simulink model "EKF_SPM_Slx2019"  (R2019a)
settings: Solver=ode45  StartTime=0.0  StopTime=0.7  MaxStep=5e-6  RelTol=1e-3
values from neighbouring files (symbols this model uses):
  alpha = 2*pi*200    (= 1256.63706144)    [EKF_SPM_settings.m]
  alphas = log(9)/t_rc    [EKF_SPM_settings.m]
  d = [-1/Ld; 0]    [EKF_SPM_settings.m]
  fpwm = 20e3    (= 20000)    [EKF_SPM_settings.m]
  gainAngle_noise = 0    [EKF_SPM_settings.m]
  gainSpeed_noise = 3.6 /60*2*pi    (= 0.376991118431)    [EKF_SPM_settings.m]
  inertia = 1.8e-4    (= 0.00018)    [EKF_SPM_settings.m]
  ivar = istdDev^2    (= 11.6508444444)    [EKF_SPM_settings.m]
  J = skewdec(2,0)    [EKF_SPM_settings.m]
  Kbs = 2/Kp_speed    [EKF_SPM_settings.m]
  ki = (-5.135 + 5.347)/Ts    (= 4240)    [EKF_SPM_settings.m]
  Ki_speed = (alphas/2/zeta)^2*inertia    [EKF_SPM_settings.m]
  kp = 5.347    [EKF_SPM_settings.m]
  Kp_speed = alphas*inertia    [EKF_SPM_settings.m]
  Ld = 3e-3    (= 0.003)    [EKF_SPM_settings.m]
  Linv = inv(L)    [EKF_SPM_settings.m]
  Lq = 3e-3    (= 0.003)    [EKF_SPM_settings.m]
  LT = 2.8    [EKF_SPM_settings.m]
  m = 3    [EKF_SPM_settings.m]
  p = 4    [EKF_SPM_settings.m]
  P0 = diag([0.1 0.1 200 10])    [EKF_SPM_settings.m]
  phi_PM = 0.1    [EKF_SPM_settings.m]
  Q = eye(4)    [EKF_SPM_settings.m]
  Qd = eye(4)    [EKF_SPM_settings.m]
  R = 1.9    [EKF_SPM_settings.m]
  R_cov = meas_sd^2*eye(2)    [EKF_SPM_settings.m]
  ramp_rate = 5    [EKF_SPM_settings.m]
  Rs = R    (= 1.9)    [EKF_SPM_settings.m]
  seed_1 = round(rand*(2^32-1))    [EKF_SPM_settings.m]
  seed_2 = round(rand*(2^32-1))    [EKF_SPM_settings.m]
  seed_4 = round(rand*(2^32-1))    [EKF_SPM_settings.m]
  seed_5 = round(rand*(2^32-1))    [EKF_SPM_settings.m]
  seed_6 = round(rand*(2^32-1))    [EKF_SPM_settings.m]
  snoise_mean = 0    [EKF_SPM_settings.m]
  snoise_std = 0.5    [EKF_SPM_settings.m]
  Ts = 1/fpwm    (= 5e-05)    [EKF_SPM_settings.m]
  Tspeed = Ts*10/10    (= 5e-05)    [EKF_SPM_settings.m]
  Vdc = 450    [EKF_SPM_settings.m]
  wm = 2*pi*ff    (= 1675.51608191)    [EKF_SPM_settings.m]
  zeta = 0.9    [EKF_SPM_settings.m]
undefined symbols (not defined in the file or in its folder): ssensor
libraries: simulink x11
(part 1 of 2)
settings Model: Creator=Nicky  LastModifiedBy=b6055800
settings DebuggingCC: ArithmeticOperatorsInVariantConditions=warning
settings CodeAppCC: StateflowObjectComments=on

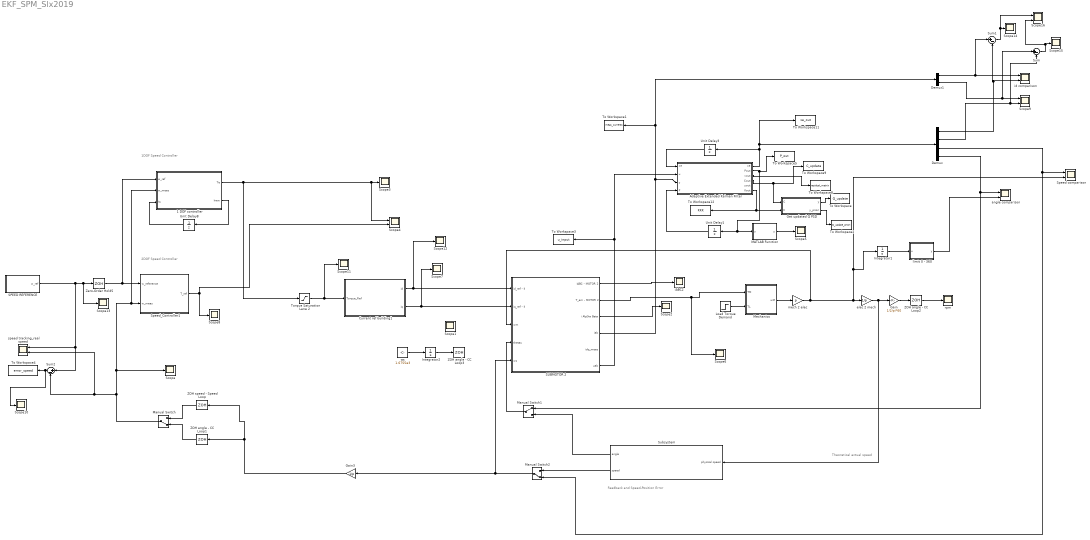
== system EKF_SPM_Slx2019 ==
  note: Theoretical actual speed
  note: Feedback and Speed-Position Error
  note: 2DOF Speed Controller
  note: 1DOF Speed Controller
  1 DOF controller : MATLAB Function  TreatAsAtomicUnit=on
  Adaptive Extended Kalman Filter : MATLAB Function  TreatAsAtomicUnit=on
  Current ref building1 : Subsystem
  Demux : Demux
  Demux1 : Demux  Outputs=2
  Gain : Gain  Gain=1/2/pi*60
  Gain3 : Gain  Gain=1/p
  Get updated Q PSD : MATLAB Function  TreatAsAtomicUnit=on
  Integrator1 : Integrator
  Integrator2 : Integrator
  Load Torque Demand : Step  Time=0.4  After=LT  SampleTime=0
  MATLAB Function : MATLAB Function  TreatAsAtomicUnit=on
  Manual Switch : ManualSwitch  CurrentSetting=0
  Manual Switch1 : ManualSwitch
  Manual Switch2 : ManualSwitch  CurrentSetting=0
  Mechanics : Subsystem
  "SPEED REFERENCE " : Subsystem
  SUBMOTOR 2 : Subsystem
  Scope{,1..3,5..8,10..15} (14 alike) : Scope
  Scope16 : Scope  NumInputPorts=2
  Scope4 : Scope  NumInputPorts=2
  Scope9 : Scope  NumInputPorts=2
  Speed comparison : Scope  NumInputPorts=2
  Speed_Controller1 : Subsystem
  Subsystem : Subsystem
  Sum : Sum  Inputs=|+-
  Sum1 : Sum  Inputs=|+-
  Sum2 : Sum  Inputs=|+-
  To Workspace : ToWorkspace  VariableName=Q_update  SaveFormat=Timeseries  SampleTime=-1
  To Workspace1 : ToWorkspace  VariableName=meas_currents  SaveFormat=Timeseries  SampleTime=-1
  To Workspace11 : ToWorkspace  VariableName=xe_out  SaveFormat=Timeseries  SampleTime=-1
  To Workspace12 : ToWorkspace  VariableName=KKK  SaveFormat=Timeseries  SampleTime=-1
  To Workspace2 : ToWorkspace  VariableName=Q_update_priori  SaveFormat=Timeseries  SampleTime=-1
  To Workspace3 : ToWorkspace  VariableName=u_input  SaveFormat=Timeseries  SampleTime=-1
  To Workspace4 : ToWorkspace  VariableName=error_speed  SaveFormat=Timeseries  SampleTime=-1
      settings: Decimation=10
  To Workspace5 : ToWorkspace  VariableName=P_out  SaveFormat=Timeseries  SampleTime=-1
  To Workspace8 : ToWorkspace  VariableName=residual_matrix  SaveFormat=Timeseries  SampleTime=-1
  To Workspace9 : ToWorkspace  VariableName=C_update  SaveFormat=Timeseries  SampleTime=-1
  Torque Saturation Lane 2 : Saturate  UpperLimit=10  LowerLimit=-10
  Unit Delay1 : UnitDelay  InitialCondition=P0  SampleTime=1/fpwm  HasFrameUpgradeWarning=on
  Unit Delay3 : UnitDelay  InitialCondition=zeros(4,1)  SampleTime=1/fpwm  HasFrameUpgradeWarning=on
  Unit Delay8 : UnitDelay  SampleTime=Ts  HasFrameUpgradeWarning=on
  ZOH angle - CC Loop1 : ZeroOrderHold  SampleTime=Ts
  ZOH angle - CC Loop2 : ZeroOrderHold  SampleTime=Ts
  ZOH angle - CC Loop3 : ZeroOrderHold  SampleTime=Ts
  ZOH speed - Speed Loop : ZeroOrderHold  SampleTime=Tspeed
  Zero-Order Hold5 : ZeroOrderHold  SampleTime=Tspeed
  angle comparison : Scope  NumInputPorts=2
  elec 2 mech : Gain  Gain=1/p
  iABC2 : Scope
  id comparison : Scope  NumInputPorts=2
  limit 0 - 360 : MATLAB Function  TreatAsAtomicUnit=on
  mech 2 elec : Gain  Gain=p
  rpm : Scope
  speed tracking_real speed : Scope  NumInputPorts=2
  ws : Constant  Value=1.6755e3
  wires:
  Mechanics/1(wM) -> mech 2 elec/1
  Load Torque Demand/1 -> Mechanics/2(TL)
  "SPEED REFERENCE "/1(w_ref) -> Scope13/1, Zero-Order Hold5/1, Sum2/1, speed tracking_real speed/1
  Sum2/1 -> Scope10/1, To Workspace4/1
  SUBMOTOR 2/1(IABC - MOTOR 2) -> iABC2/1
  Manual Switch/1 -> speed tracking_real speed/2, Sum2/2, Speed_Controller1/2(w_meas), 1 DOF controller/2(w_meas), Scope/1
  1 DOF controller/1(Te) -> Torque Saturation Lane 2/1, Scope4/1, Scope3/1
  Zero-Order Hold5/1 -> Speed_Controller1/1(w_reference), 1 DOF controller/1(w_ref)
  Torque Saturation Lane 2/1 -> Scope11/1, Current ref building1/1(Torque_Ref)
  SUBMOTOR 2/3(i Alp[ha Beta) -> Scope2/1
  Gain/1 -> ZOH angle - CC Loop2/1
  elec 2 mech/1 -> Subsystem/1(physical speed), Gain/1
  ZOH angle - CC Loop2/1 -> rpm/1
  Unit Delay8/1 -> 1 DOF controller/3(Iw)
  1 DOF controller/2(Inew) -> Unit Delay8/1
  Speed_Controller1/1(T_ref) -> Scope8/1, Scope4/2
  Unit Delay1/1 -> Adaptive Extended Kalman Filter/4(P)
  Unit Delay3/1 -> Adaptive Extended Kalman Filter/1("xe ")
  Demux/1 -> Sum1/2, id comparison/2
  Demux/2 -> Sum/2, Scope9/2
  Demux1/1 -> Sum1/1, id comparison/1
  Demux1/2 -> Sum/1, Scope9/1
  Integrator1/1 -> limit 0 - 360/1(u)
  MATLAB Function/1(y) -> Scope5/1
  Manual Switch2/1 -> SUBMOTOR 2/5(ws), Gain3/1
  ZOH angle - CC Loop1/1 -> Manual Switch/2
  ZOH speed - Speed Loop/1 -> Manual Switch/1
  SUBMOTOR 2/2(T_em - MOTOR 2) -> Scope6/1, Mechanics/1(TM)
  Integrator2/1 -> ZOH angle - CC Loop3/1
  ws/1 -> Integrator2/1
  Current ref building1/1(id) -> Scope12/1, SUBMOTOR 2/1(id_ref - II)
  Current ref building1/2(iq) -> Scope7/1, SUBMOTOR 2/2(iq_ref - II)
  SUBMOTOR 2/4(iab) -> Demux1/1, To Workspace1/1, Adaptive Extended Kalman Filter/3(y)
  SUBMOTOR 2/6("uab ") -> To Workspace3/1, Adaptive Extended Kalman Filter/2(u)
  Demux/4 -> Manual Switch1/1, angle comparison/1
  Subsystem/1(angle) -> Manual Switch1/2
  Manual Switch1/1 -> SUBMOTOR 2/4(thetas)
  Subsystem/2(speed) -> Manual Switch2/1
  Demux/3 -> Manual Switch2/2, Speed comparison/1
  Gain3/1 -> ZOH speed - Speed Loop/1, ZOH angle - CC Loop1/1
  mech 2 elec/1 -> Speed comparison/2, Integrator1/1, elec 2 mech/1, SUBMOTOR 2/3(wm)
  Adaptive Extended Kalman Filter/2(Pout) -> To Workspace5/1, MATLAB Function/1(u), Unit Delay1/1
  Adaptive Extended Kalman Filter/3(vout) -> To Workspace8/1
  Adaptive Extended Kalman Filter/4(Cout) -> Get updated Q PSD/1(C), To Workspace9/1
  Adaptive Extended Kalman Filter/1(xe) -> To Workspace11/1, Demux/1, Unit Delay3/1
  Adaptive Extended Kalman Filter/6(Kout) -> Get updated Q PSD/2(K), To Workspace12/1
  Sum1/1 -> Scope16/1, Scope14/1
  Sum/1 -> Scope16/2, Scope15/1
  Get updated Q PSD/1(y) -> To Workspace/1
  Get updated Q PSD/2(y_priori) -> To Workspace2/1
  limit 0 - 360/1(y) -> angle comparison/2

== system EKF_SPM_Slx2019/Current ref building1 ==
  note: THIS BLOCK COULD IMPLEMENT A LOOKUP TABLE, AND OR ANY FLUX WEAKENING REFERENCING FOR OPTIMUM CURRENTS GIVEN A SPECIFIC TORQUE
  Torque_Ref : Inport
  Demux : Demux  Outputs=2
  IPM : MATLAB Function  TreatAsAtomicUnit=on
  Manual Switch : ManualSwitch
  Mux : Mux  Inputs=2
  Mux1 : Mux  Inputs=2
  SPM-current reference : MATLAB Function  TreatAsAtomicUnit=on
  To Workspace : ToWorkspace  VariableName=Iref_magnitude_MTPA  SaveFormat=Timeseries  SampleTime=-1
      settings: Decimation=10
  To Workspace1 : ToWorkspace  VariableName=Iref_magnitude_SPM  SaveFormat=Timeseries  SampleTime=-1
      settings: Decimation=10
  id : Outport
  iq : Outport  Port=2
  wires:
  SPM-current reference/1(id) -> Mux1/1
  SPM-current reference/2(iq) -> Mux1/2
  Demux/1 -> id/1
  Demux/2 -> iq/1
  Manual Switch/1 -> Demux/1
  IPM/2(iq) -> Mux/2
  IPM/1(id) -> Mux/1
  Mux1/1 -> Manual Switch/1
  Mux/1 -> Manual Switch/2
  IPM/3(Imag) -> To Workspace/1
  SPM-current reference/3(Imag) -> To Workspace1/1
  Torque_Ref/1 -> IPM/1(Tref), SPM-current reference/1(T_ref)

== system EKF_SPM_Slx2019/Mechanics ==
  TM : Inport
  TL : Inport  Port=2
  Gain : Gain  Gain=1/inertia  SaturateOnIntegerOverflow=on  OutDataTypeStr=Inherit: Same as input  ParamDataTypeStr=Inherit: Same as input
  Integrator : Integrator
  Sum : Sum  Inputs=|+-  SaturateOnIntegerOverflow=on  InputSameDT=on  OutDataTypeStr=Inherit: Same as first input
  wM : Outport
  wires:
  TL/1 -> Sum/2
  Sum/1 -> Gain/1
  Gain/1 -> Integrator/1
  Integrator/1 -> wM/1
  TM/1 -> Sum/1

== system EKF_SPM_Slx2019/SPEED REFERENCE  ==
  Constant : Constant  Value=0
  Go Down : simulink/Sources/Ramp  slope=-ramp_rate*wm/p  start=0.5  InitialOutput=0
  Go Flat : simulink/Sources/Ramp  slope=-ramp_rate*wm/p  start=1/ramp_rate  InitialOutput=0
  Go Flat2 : simulink/Sources/Ramp  slope=ramp_rate*wm/p  start=0.5+1/ramp_rate  InitialOutput=0
  Manual Switch : ManualSwitch  CurrentSetting=0
  Manual Switch1 : ManualSwitch
  Manual Switch2 : ManualSwitch
  Ramp Up : simulink/Sources/Ramp  slope=ramp_rate*wm/p  start=0  InitialOutput=0
  Step : Step  Time=0.05  After=wm/p  SampleTime=0
  Sum : Sum  Inputs=|++++
  w_ref : Outport
  wires:
  Ramp Up/1 -> Sum/1
  Step/1 -> Manual Switch/1
  Manual Switch/1 -> w_ref/1
  Sum/1 -> Manual Switch/2
  Go Flat/1 -> Sum/2
  Manual Switch1/1 -> Sum/3
  Go Down/1 -> Manual Switch1/2
  Constant/1 -> Manual Switch2/1, Manual Switch1/1
  Go Flat2/1 -> Manual Switch2/2
  Manual Switch2/1 -> Sum/4

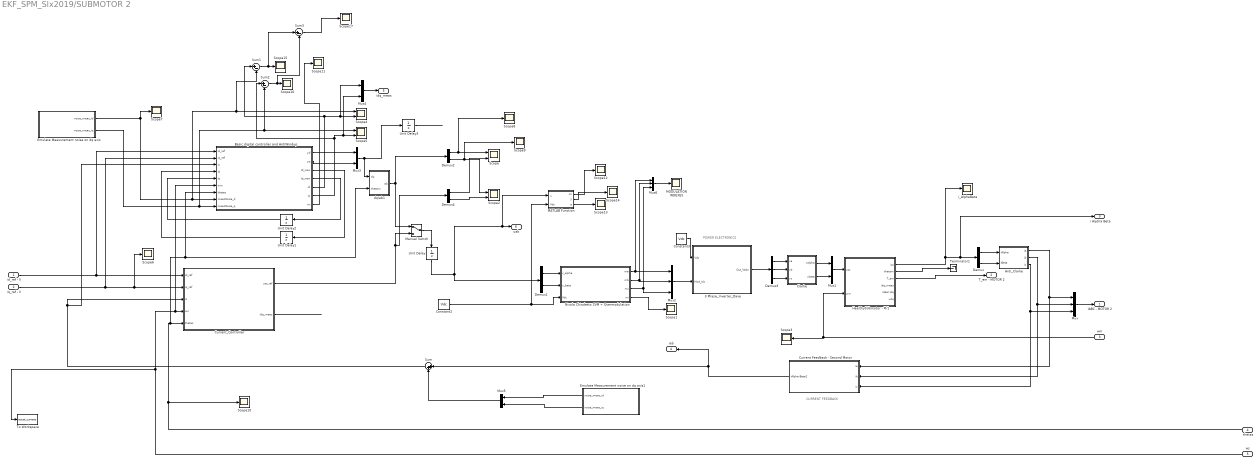
== system EKF_SPM_Slx2019/SUBMOTOR 2 ==
  note: CURRENT FEEDBACK
  note: POWER ELECTRONICS
  id_ref - II : Inport
  iq_ref - II : Inport  Port=2
  wm : Inport  Port=3
  thetas : Inport  Port=4
  ws : Inport  Port=5
  3 Phase_Inverter_Dave : Subsystem
  Anti_Clarke : Subsystem
  Basic digital controller and AntiWindup : MATLAB Function  TreatAsAtomicUnit=on
  Clarke : Subsystem
  Constant2 : Constant  Value=Vdc
  Constant3 : Constant  Value=Vdc
  Current Feedback - Second Motor : Subsystem
  Current_Controller : Subsystem
  Demux{,1..2,4} (4 alike) : Demux  Outputs=2
  Demux3 : Demux  Outputs=3
  Emulate Measurement noise on dq axis : Subsystem
  Emulate Measurement noise on dq axis1 : Subsystem
  HealthySUbmotor - PI/1 : Subsystem
  MATLAB Function : MATLAB Function  TreatAsAtomicUnit=on
  MODULATION INDEXES : Scope
  Manual Switch : ManualSwitch
  Mux : Mux  Inputs=3
  Mux{1,3..5} (4 alike) : Mux  Inputs=2
  Mux2 : Mux  Inputs=3
  Mux6 : Mux  Inputs=3
  Nicola Chiodetto SVM + Overmodulation : MATLAB Function  TreatAsAtomicUnit=on
  Scope{,2,4..5} (4 alike) : Scope  NumInputPorts=2
  Scope{1,3,6..17} (14 alike) : Scope
  Sum : Sum  Inputs=|++
  Sum1 : Sum  Inputs=|+-
  Sum2 : Sum  Inputs=|+-
  Sum3 : Sum  Inputs=|+-
  Terminator1 : Terminator
  To Workspace : ToWorkspace  VariableName=actual_currents  SaveFormat=Timeseries  SampleTime=-1
  Unit Delay{,1..3} (4 alike) : UnitDelay  SampleTime=1/fpwm  HasFrameUpgradeWarning=on
  dq/ab1 : Subsystem
  i_AlphaBeta : Scope
  IABC - MOTOR 2 : Outport
  T_em - MOTOR 2 : Outport  Port=2
  i Alp[ha Beta : Outport  Port=3
  iab : Outport  Port=4
  idq_meas : Outport  Port=5
  "uab " : Outport  Port=6
  wires:
  HealthySUbmotor - PI/1/1(iss) -> Demux/1, i Alp[ha Beta/1, i_AlphaBeta/1
  Anti_Clarke/3(ic) -> Current Feedback - Second Motor/3(ic), Mux/3
  Demux3/1 -> Clarke/1(va)
  Clarke/2(vbeta) -> Mux1/2
  iq_ref - II/1 -> Basic digital controller and AntiWindup/2(iq_ref), Current_Controller/2(iq_ref), Scope6/1
  Clarke/1(valpha) -> Mux1/1
  Demux/2 -> Anti_Clarke/2(iBeta)
  Current_Controller/1(uss_ref) -> Demux4/1, Manual Switch/2
  Anti_Clarke/2(ib) -> Current Feedback - Second Motor/2(ib), Mux/2
  Constant3/1 -> 3 Phase_Inverter_Dave/1(Vdc)
  ws/1 -> Basic digital controller and AntiWindup/6(wm), Current_Controller/4(ws), To Workspace/1
  Demux/1 -> Anti_Clarke/1(iAlpha)
  Demux3/2 -> Clarke/2(vb)
  Mux2/1 -> 3 Phase_Inverter_Dave/2(Mod_Idx)
  HealthySUbmotor - PI/1/2(thetam) -> Terminator1/1
  Mux6/1 -> MODULATION INDEXES/1
  Demux1/1 -> Nicola Chiodetto SVM + Overmodulation/1(v_alpha)
  Demux1/2 -> Nicola Chiodetto SVM + Overmodulation/2(v_beta)
  Demux3/3 -> Clarke/3(vc)
  Nicola Chiodetto SVM + Overmodulation/4(mi) -> Scope1/1
  HealthySUbmotor - PI/1/3(T_em) -> T_em - MOTOR 2/1
  wm/1 -> HealthySUbmotor - PI/1/2(wm), Scope3/1
  Nicola Chiodetto SVM + Overmodulation/1(ma) -> Mux2/1, Mux6/1
  Mux/1 -> IABC - MOTOR 2/1
  Nicola Chiodetto SVM + Overmodulation/2(mb) -> Mux2/2, Mux6/2
  Nicola Chiodetto SVM + Overmodulation/3(mc) -> Mux2/3, Mux6/3
  Current Feedback - Second Motor/1(iAlpha-Beta2) -> iab/1, Sum/1
  Anti_Clarke/1(ia) -> Current Feedback - Second Motor/1(ia), Mux/1
  Mux1/1 -> HealthySUbmotor - PI/1/1(uss)
  3 Phase_Inverter_Dave/1(Out_Vabc) -> Demux3/1
  Basic digital controller and AntiWindup/1(yd) -> Mux3/1
  Basic digital controller and AntiWindup/2(yq) -> Mux3/2
  Mux3/1 -> Unit Delay3/1, dq/ab1/1(dq)
  Basic digital controller and AntiWindup/3(Id_new) -> Unit Delay1/1
  Unit Delay1/1 -> Basic digital controller and AntiWindup/4(Id)
  Basic digital controller and AntiWindup/4(Iq_new) -> Unit Delay2/1
  Unit Delay2/1 -> Basic digital controller and AntiWindup/5(Iq)
  id_ref - II/1 -> Basic digital controller and AntiWindup/1(id_ref), Current_Controller/1(id_ref)
  dq/ab1/1(ab) -> Demux2/1, Manual Switch/1
  Manual Switch/1 -> Unit Delay/1
  Demux2/1 -> Scope8/1, Scope/1
  Demux4/1 -> Scope/2
  Demux2/2 -> Scope9/1, Scope2/1
  Demux4/2 -> Scope2/2
  thetas/1 -> Scope10/1, dq/ab1/2(thetam), Basic digital controller and AntiWindup/7(thetas), Current_Controller/5(thetas)
  Basic digital controller and AntiWindup/5(id) -> Sum1/1, Mux4/1, Scope4/2
  Basic digital controller and AntiWindup/6(iq) -> Sum2/1, Mux4/2, Scope5/2
  Current_Controller/2(idq_meas) -> ?
  Emulate Measurement noise on dq axis/1(noise_meas_id) -> Scope7/1, Sum1/2, Scope4/1, Basic digital controller and AntiWindup/8(measNoise_d)
  Mux4/1 -> idq_meas/1
  Emulate Measurement noise on dq axis/2(noise_meas_iq) -> Sum2/2, Scope5/1, Basic digital controller and AntiWindup/9(measNoise_q)
  Unit Delay3/1 -> ?
  Emulate Measurement noise on dq axis1/1(noise_meas_id) -> Mux5/1
  Emulate Measurement noise on dq axis1/2(noise_meas_iq) -> Mux5/2
  Sum/1 -> Basic digital controller and AntiWindup/3(is), Current_Controller/3(is)
  Mux5/1 -> Sum/2
  Unit Delay/1 -> Demux1/1, MATLAB Function/1(u), "uab "/1
  Constant2/1 -> MATLAB Function/2(Vdc), Nicola Chiodetto SVM + Overmodulation/3(Vdc)
  Basic digital controller and AntiWindup/7(mi) -> Scope11/1
  MATLAB Function/1(mi) -> Scope12/1
  MATLAB Function/3(a) -> Scope13/1
  MATLAB Function/2(y) -> Scope14/1
  Sum1/1 -> Sum3/1, Scope15/1
  Sum2/1 -> Sum3/2, Scope16/1
  Sum3/1 -> Scope17/1

== system EKF_SPM_Slx2019/Speed_Controller1 ==
  w_reference : Inport
  w_meas : Inport  Port=2
  Check_AdvancedFF : MATLAB Function  TreatAsAtomicUnit=on
  Scope : Scope
  Scope2 : Scope
  Terminator : Terminator
  Unit Delay{4..8} (5 alike) : UnitDelay  SampleTime=Tspeed  HasFrameUpgradeWarning=on
  T_ref : Outport
  wires:
  Unit Delay6/1 -> Check_AdvancedFF/5(I)
  Unit Delay8/1 -> Check_AdvancedFF/7(Tffn_2)
  Unit Delay5/1 -> Check_AdvancedFF/3(wn_2)
  w_reference/1 -> Check_AdvancedFF/1(w_ref), Unit Delay4/1
  Check_AdvancedFF/3(Tffn) -> Unit Delay7/1
  Unit Delay4/1 -> Unit Delay5/1, Check_AdvancedFF/2(wn_1)
  Check_AdvancedFF/2(Inew) -> Unit Delay6/1, Scope2/1
  Unit Delay7/1 -> Unit Delay8/1, Check_AdvancedFF/6(Tffn_1)
  Check_AdvancedFF/1(Te) -> Scope/1, T_ref/1
  w_meas/1 -> Check_AdvancedFF/4(w_meas)
  Check_AdvancedFF/4(sat) -> Terminator/1

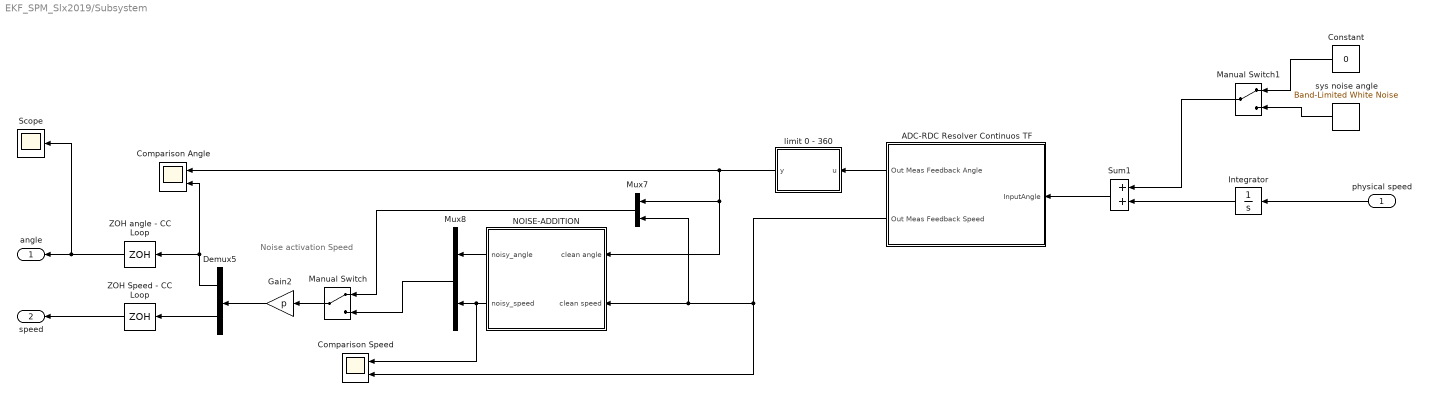
== system EKF_SPM_Slx2019/Subsystem ==
  note: Noise activation Speed
  physical speed : Inport
  ADC-RDC Resolver Continuos TF : Subsystem  mask{a=ssensor.a, b=ssensor.b, c=ssensor.c, t=ssensor.t, k1=ssensor.k1, k2=ssensor.k2}
      mask prompts: a "Comp zero coefficienc"; b "Comp pole coeff"; c "Int gain"; t "sample period"; k1 "ADC gain"; k2 "Error gain"
  Comparison Angle : Scope  NumInputPorts=2
  Comparison Speed : Scope  NumInputPorts=2
  Constant : Constant  Value=0
  Demux5 : Demux  Outputs=2
  Gain2 : Gain  Gain=p
  Integrator : Integrator
  Manual Switch : ManualSwitch
  Manual Switch1 : ManualSwitch
  Mux7 : Mux  Inputs=2
  Mux8 : Mux  Inputs=2
  NOISE-ADDITION : Subsystem
  Scope : Scope
  Sum1 : Sum
  ZOH Speed - CC Loop : ZeroOrderHold  SampleTime=Ts
  ZOH angle - CC Loop : ZeroOrderHold  SampleTime=Ts
  limit 0 - 360 : MATLAB Function  TreatAsAtomicUnit=on
  sys noise angle : simulink/Sources/Band-Limited White Noise  Cov=[Q(4,4)*Ts]  Ts=Ts  seed=[seed_6]
  angle : Outport
  speed : Outport  Port=2
  wires:
  Mux7/1 -> Manual Switch/1
  Mux8/1 -> Manual Switch/2
  Gain2/1 -> Demux5/1
  Manual Switch/1 -> Gain2/1
  physical speed/1 -> Integrator/1
  Demux5/1 -> Comparison Angle/2, ZOH angle - CC Loop/1
  Demux5/2 -> ZOH Speed - CC Loop/1
  NOISE-ADDITION/1(noisy_angle) -> Mux8/1
  NOISE-ADDITION/2(noisy_speed) -> Comparison Speed/1, Mux8/2
  ZOH Speed - CC Loop/1 -> speed/1
  Integrator/1 -> Sum1/2
  Manual Switch1/1 -> Sum1/1
  sys noise angle/1 -> Manual Switch1/2
  Constant/1 -> Manual Switch1/1
  ZOH angle - CC Loop/1 -> Scope/1, angle/1
  ADC-RDC Resolver Continuos TF/1(Out Meas Feedback Angle) -> limit 0 - 360/1(u)
  ADC-RDC Resolver Continuos TF/2(Out Meas Feedback Speed) -> Comparison Speed/2, Mux7/2, NOISE-ADDITION/2(clean speed)
  Sum1/1 -> ADC-RDC Resolver Continuos TF/1(InputAngle)
  limit 0 - 360/1(y) -> Comparison Angle/1, NOISE-ADDITION/1(clean angle), Mux7/1

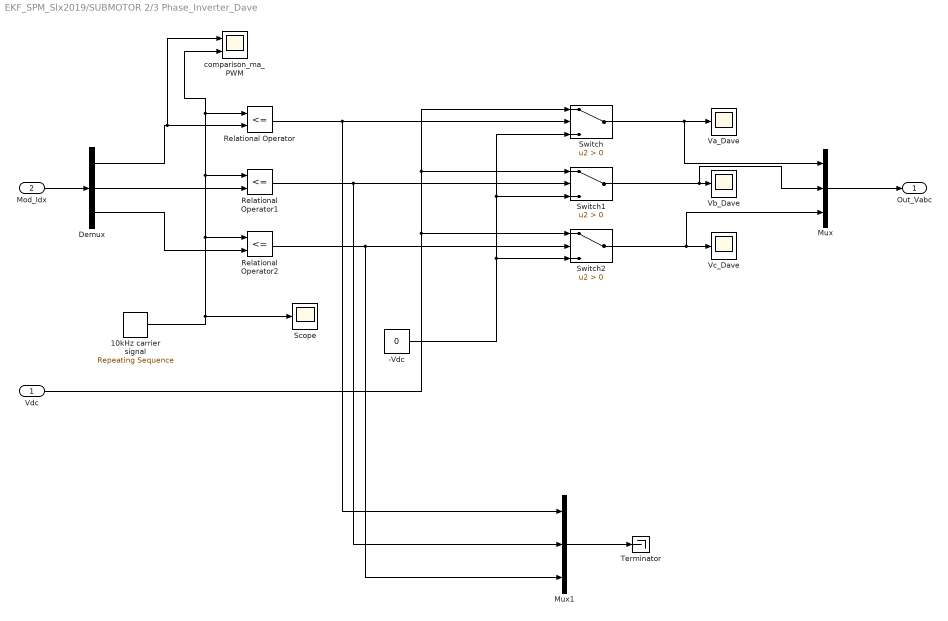
== system EKF_SPM_Slx2019/SUBMOTOR 2/3 Phase_Inverter_Dave ==
  Vdc : Inport
  Mod_Idx : Inport  Port=2
  -Vdc : Constant  Value=0
  10kHz carrier signal : simulink/Sources/Repeating Sequence  rep_seq_t=[0 .5*Ts Ts]  rep_seq_y="[1  0 1]"
  Demux : Demux  Outputs=3
  Mux : Mux  Inputs=3
  Mux1 : Mux  Inputs=3
  Relational Operator : RelationalOperator  Operator=<=  OutDataTypeStr=boolean  RndMeth=Nearest
  Relational Operator1 : RelationalOperator  Operator=<=  OutDataTypeStr=boolean  RndMeth=Nearest
  Relational Operator2 : RelationalOperator  Operator=<=  OutDataTypeStr=boolean  RndMeth=Nearest
  Scope : Scope
  Switch : Switch  Criteria=u2 > Threshold
  Switch1 : Switch  Criteria=u2 > Threshold
  Switch2 : Switch  Criteria=u2 > Threshold
  Terminator : Terminator
  Va_Dave : Scope
  Vb_Dave : Scope
  Vc_Dave : Scope
  comparison_ma_PWM : Scope  NumInputPorts=2
  Out_Vabc : Outport
  wires:
  Vdc/1 -> Switch2/1, Switch1/1, Switch/1
  -Vdc/1 -> Switch2/3, Switch1/3, Switch/3
  Switch/1 -> Mux/1, Va_Dave/1
  Switch2/1 -> Mux/3, Vc_Dave/1
  Relational Operator2/1 -> Mux1/3, Switch2/2
  Relational Operator1/1 -> Mux1/2, Switch1/2
  10kHz carrier signal/1 -> Scope/1, Relational Operator1/1, comparison_ma_PWM/2, Relational Operator/1, Relational Operator2/1
  Demux/1 -> comparison_ma_PWM/1, Relational Operator/2
  Mod_Idx/1 -> Demux/1
  Demux/3 -> Relational Operator2/2
  Demux/2 -> Relational Operator1/2
  Relational Operator/1 -> Mux1/1, Switch/2
  Mux/1 -> Out_Vabc/1
  Switch1/1 -> Mux/2, Vb_Dave/1
  Mux1/1 -> Terminator/1

== system EKF_SPM_Slx2019/SUBMOTOR 2/Anti_Clarke ==
  iAlpha : Inport
  iBeta : Inport  Port=2
  " root3/2" : Gain  Gain=0.86602540378443864676372317075294  SaturateOnIntegerOverflow=on  OutDataTypeStr=Inherit: Same as input  ParamDataTypeStr=Inherit: Same as input
  1/2 : Gain  Gain=1/2  SaturateOnIntegerOverflow=on  OutDataTypeStr=Inherit: Same as input  ParamDataTypeStr=Inherit: Same as input
  Sum2 : Sum  Inputs=--  SaturateOnIntegerOverflow=on  InputSameDT=on  OutDataTypeStr=Inherit: Same as first input
  Sum4 : Sum  Inputs=-+  SaturateOnIntegerOverflow=on  InputSameDT=on  OutDataTypeStr=Inherit: Same as first input
  ia : Outport
  ib : Outport  Port=2
  ic : Outport  Port=3
  wires:
  iBeta/1 -> " root3/2"/1
  " root3/2"/1 -> Sum4/2, Sum2/2
  1/2/1 -> Sum2/1, Sum4/1
  Sum2/1 -> ic/1
  Sum4/1 -> ib/1
  iAlpha/1 -> 1/2/1, ia/1

== system EKF_SPM_Slx2019/SUBMOTOR 2/Clarke ==
  va : Inport
  vb : Inport  Port=2
  vc : Inport  Port=3
  " " : Gain  Gain=2/3  SaturateOnIntegerOverflow=on  OutDataTypeStr=Inherit: Same as input  ParamDataTypeStr=Inherit: Same as input
  "   " : Gain  Gain=1/3  SaturateOnIntegerOverflow=on  OutDataTypeStr=Inherit: Same as input  ParamDataTypeStr=Inherit: Same as input
  "    " : Gain  Gain=1/3  SaturateOnIntegerOverflow=on  OutDataTypeStr=Inherit: Same as input  ParamDataTypeStr=Inherit: Same as input
  " 1/root3" : Gain  Gain=0.57735026918962576450914878050196  SaturateOnIntegerOverflow=on  OutDataTypeStr=Inherit: Same as input  ParamDataTypeStr=Inherit: Same as input
  Sum1 : Sum  Inputs=+-  SaturateOnIntegerOverflow=on  InputSameDT=on  OutDataTypeStr=Inherit: Same as first input
  Sum4 : Sum  Inputs=+--  SaturateOnIntegerOverflow=on  InputSameDT=on  OutDataTypeStr=Inherit: Same as first input
  valpha : Outport
  vbeta : Outport  Port=2
  wires:
  Sum4/1 -> valpha/1
  " "/1 -> Sum4/1
  va/1 -> " "/1
  "    "/1 -> Sum4/2
  "   "/1 -> Sum4/3
  vb/1 -> "    "/1, Sum1/1
  vc/1 -> "   "/1, Sum1/2
  Sum1/1 -> " 1/root3"/1
  " 1/root3"/1 -> vbeta/1

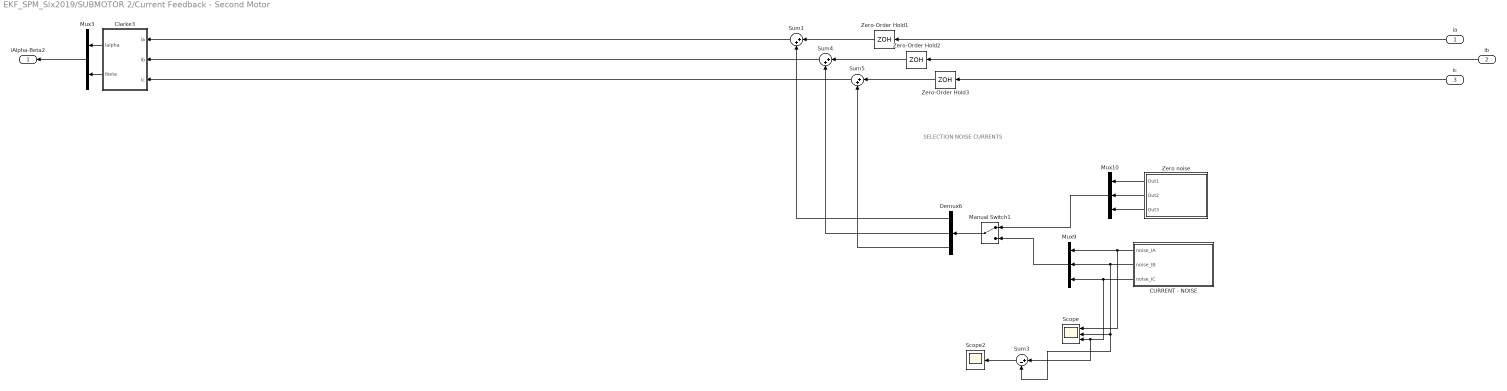
== system EKF_SPM_Slx2019/SUBMOTOR 2/Current Feedback - Second Motor ==
  note: SELECTION NOISE CURRENTS
  ia : Inport
  ib : Inport  Port=2
  ic : Inport  Port=3
  CURRENT - NOISE : Subsystem
  Clarke3 : Subsystem
  Demux6 : Demux  Outputs=3
  Manual Switch1 : ManualSwitch
  Mux10 : Mux  Inputs=3
  Mux3 : Mux  Inputs=2
  Mux9 : Mux  Inputs=3
  Scope : Scope  NumInputPorts=3
  Scope2 : Scope
  Sum1 : Sum  Inputs=|++
  Sum3 : Sum  Inputs=|+-
  Sum4 : Sum  Inputs=|++
  Sum5 : Sum  Inputs=|++
  Zero noise : Subsystem
  Zero-Order Hold1 : ZeroOrderHold  SampleTime=1/fpwm
  Zero-Order Hold2 : ZeroOrderHold  SampleTime=1/fpwm
  Zero-Order Hold3 : ZeroOrderHold  SampleTime=1/fpwm
  iAlpha-Beta2 : Outport
  wires:
  Sum3/1 -> Scope2/1
  CURRENT - NOISE/1(noise_IA) -> Mux9/1, Scope/1
  Clarke3/1(ialpha) -> Mux3/1
  Demux6/3 -> Sum5/2
  Zero-Order Hold3/1 -> Sum5/1
  Sum4/1 -> Clarke3/2(ib)
  Zero-Order Hold1/1 -> Sum1/1
  Zero-Order Hold2/1 -> Sum4/1
  Mux3/1 -> iAlpha-Beta2/1
  CURRENT - NOISE/2(noise_IB) -> Mux9/2, Sum3/2, Scope/2
  Zero noise/1(Out1) -> Mux10/1
  ia/1 -> Zero-Order Hold1/1
  Sum5/1 -> Clarke3/3(ic)
  Zero noise/2(Out2) -> Mux10/2
  Zero noise/3(Out3) -> Mux10/3
  Mux9/1 -> Manual Switch1/2
  Demux6/1 -> Sum1/2
  Manual Switch1/1 -> Demux6/1
  Mux10/1 -> Manual Switch1/1
  Demux6/2 -> Sum4/2
  CURRENT - NOISE/3(noise_IC) -> Mux9/3, Sum3/1, Scope/3
  Clarke3/2(ibeta) -> Mux3/2
  ib/1 -> Zero-Order Hold2/1
  ic/1 -> Zero-Order Hold3/1
  Sum1/1 -> Clarke3/1(ia)

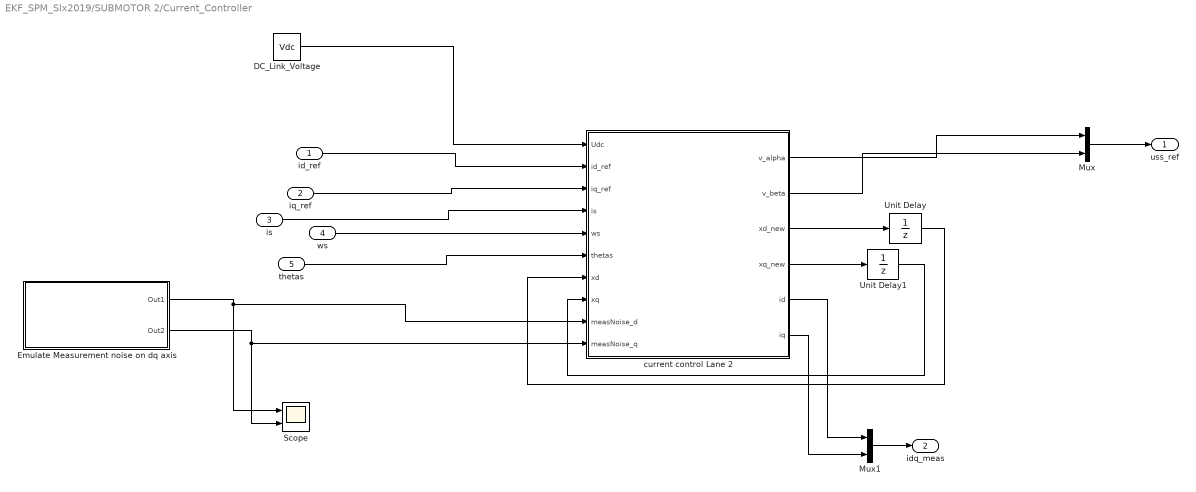
== system EKF_SPM_Slx2019/SUBMOTOR 2/Current_Controller ==
  id_ref : Inport
  iq_ref : Inport  Port=2
  is : Inport  Port=3
  ws : Inport  Port=4
  thetas : Inport  Port=5
  DC_Link_Voltage : Constant  Value=Vdc
  Emulate Measurement noise on dq axis : Subsystem
  Mux : Mux  Inputs=2
  Mux1 : Mux  Inputs=2
  Scope : Scope  NumInputPorts=2
  Unit Delay : UnitDelay  SampleTime=Ts  HasFrameUpgradeWarning=on
  Unit Delay1 : UnitDelay  SampleTime=Ts  HasFrameUpgradeWarning=on
  current control Lane 2 : MATLAB Function  TreatAsAtomicUnit=on
  uss_ref : Outport
  idq_meas : Outport  Port=2
  wires:
  id_ref/1 -> current control Lane 2/2(id_ref)
  is/1 -> current control Lane 2/4(is)
  DC_Link_Voltage/1 -> current control Lane 2/1(Udc)
  iq_ref/1 -> current control Lane 2/3(iq_ref)
  thetas/1 -> current control Lane 2/6(thetas)
  Unit Delay/1 -> current control Lane 2/7(xd)
  ws/1 -> current control Lane 2/5(ws)
  Unit Delay1/1 -> current control Lane 2/8(xq)
  current control Lane 2/4(xq_new) -> Unit Delay1/1
  current control Lane 2/3(xd_new) -> Unit Delay/1
  Mux/1 -> uss_ref/1
  current control Lane 2/2(v_beta) -> Mux/2
  current control Lane 2/1(v_alpha) -> Mux/1
  Emulate Measurement noise on dq axis/1(Out1) -> Scope/1, current control Lane 2/9(measNoise_d)
  Emulate Measurement noise on dq axis/2(Out2) -> Scope/2, current control Lane 2/10(measNoise_q)
  current control Lane 2/5(id) -> Mux1/1
  Mux1/1 -> idq_meas/1
  current control Lane 2/6(iq) -> Mux1/2

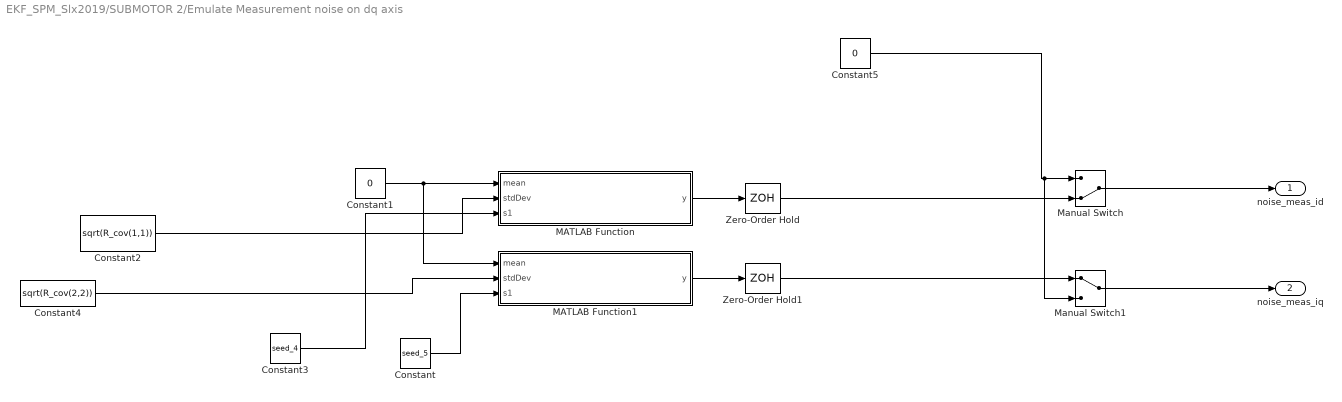
== system EKF_SPM_Slx2019/SUBMOTOR 2/Emulate Measurement noise on dq axis ==
  Constant : Constant  Value=seed_5
  Constant1 : Constant  Value=0
  Constant2 : Constant  Value=sqrt(R_cov(1,1))
  Constant3 : Constant  Value=seed_4
  Constant4 : Constant  Value=sqrt(R_cov(2,2))
  Constant5 : Constant  Value=0
  MATLAB Function : MATLAB Function  TreatAsAtomicUnit=on
  MATLAB Function1 : MATLAB Function  TreatAsAtomicUnit=on
  Manual Switch : ManualSwitch  CurrentSetting=0
  Manual Switch1 : ManualSwitch
  Zero-Order Hold : ZeroOrderHold  SampleTime=Ts
  Zero-Order Hold1 : ZeroOrderHold  SampleTime=Ts
  noise_meas_id : Outport
  noise_meas_iq : Outport  Port=2
  wires:
  Constant1/1 -> MATLAB Function1/1(mean), MATLAB Function/1(mean)
  Constant3/1 -> MATLAB Function/3(s1)
  Constant/1 -> MATLAB Function1/3(s1)
  Constant4/1 -> MATLAB Function1/2(stdDev)
  MATLAB Function/1(y) -> Zero-Order Hold/1
  MATLAB Function1/1(y) -> Zero-Order Hold1/1
  Constant2/1 -> MATLAB Function/2(stdDev)
  Constant5/1 -> Manual Switch1/2, Manual Switch/1
  Zero-Order Hold/1 -> Manual Switch/2
  Manual Switch/1 -> noise_meas_id/1
  Zero-Order Hold1/1 -> Manual Switch1/1
  Manual Switch1/1 -> noise_meas_iq/1

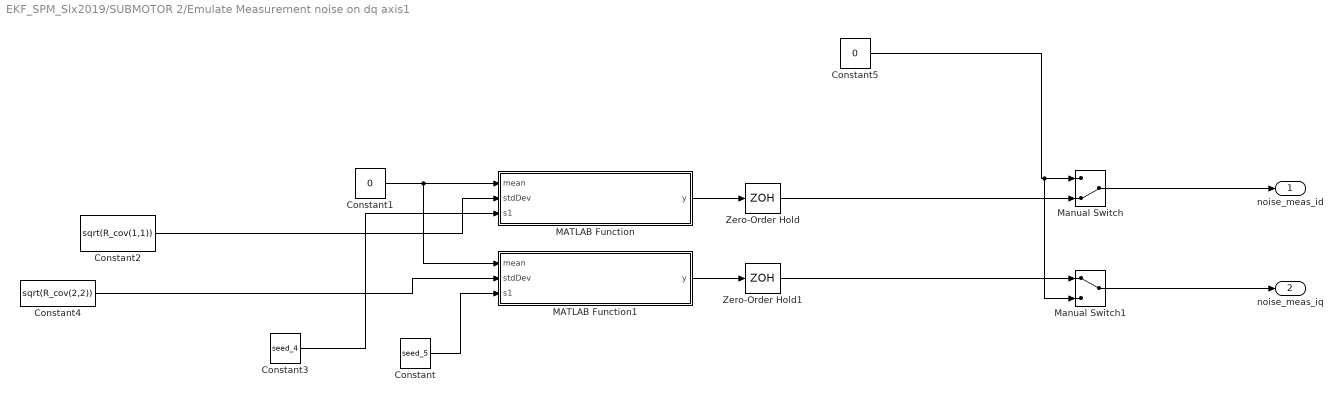
== system EKF_SPM_Slx2019/SUBMOTOR 2/Emulate Measurement noise on dq axis1 ==
  Constant : Constant  Value=seed_5
  Constant1 : Constant  Value=0
  Constant2 : Constant  Value=sqrt(R_cov(1,1))
  Constant3 : Constant  Value=seed_4
  Constant4 : Constant  Value=sqrt(R_cov(2,2))
  Constant5 : Constant  Value=0
  MATLAB Function : MATLAB Function  TreatAsAtomicUnit=on
  MATLAB Function1 : MATLAB Function  TreatAsAtomicUnit=on
  Manual Switch : ManualSwitch  CurrentSetting=0
  Manual Switch1 : ManualSwitch
  Zero-Order Hold : ZeroOrderHold  SampleTime=Ts
  Zero-Order Hold1 : ZeroOrderHold  SampleTime=Ts
  noise_meas_id : Outport
  noise_meas_iq : Outport  Port=2
  wires:
  Constant1/1 -> MATLAB Function1/1(mean), MATLAB Function/1(mean)
  Constant3/1 -> MATLAB Function/3(s1)
  Constant/1 -> MATLAB Function1/3(s1)
  Constant4/1 -> MATLAB Function1/2(stdDev)
  MATLAB Function/1(y) -> Zero-Order Hold/1
  MATLAB Function1/1(y) -> Zero-Order Hold1/1
  Constant2/1 -> MATLAB Function/2(stdDev)
  Constant5/1 -> Manual Switch1/2, Manual Switch/1
  Zero-Order Hold/1 -> Manual Switch/2
  Manual Switch/1 -> noise_meas_id/1
  Zero-Order Hold1/1 -> Manual Switch1/1
  Manual Switch1/1 -> noise_meas_iq/1

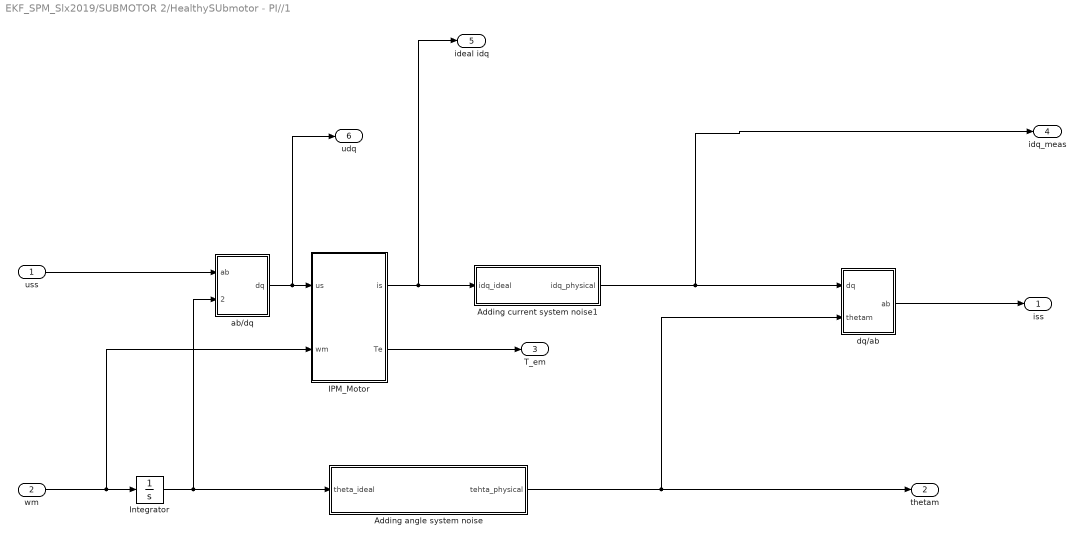
== system EKF_SPM_Slx2019/SUBMOTOR 2/HealthySUbmotor - PI//1 ==
  uss : Inport
  wm : Inport  Port=2
  Adding angle system noise : Subsystem
  Adding current system noise1 : Subsystem
  IPM_Motor : Subsystem
  Integrator : Integrator
  ab/dq : Subsystem
  dq/ab : Subsystem
  iss : Outport
  thetam : Outport  Port=2
  T_em : Outport  Port=3
  idq_meas : Outport  Port=4
  ideal idq : Outport  Port=5
  udq : Outport  Port=6
  wires:
  uss/1 -> ab/dq/1(ab)
  dq/ab/1(ab) -> iss/1
  IPM_Motor/2(Te) -> T_em/1
  ab/dq/1(dq) -> udq/1, IPM_Motor/1(us)
  wm/1 -> IPM_Motor/2(wm), Integrator/1
  IPM_Motor/1(is) -> Adding current system noise1/1(idq_ideal), ideal idq/1
  Integrator/1 -> ab/dq/2(thetame), Adding angle system noise/1(theta_ideal)
  Adding angle system noise/1(tehta_physical) -> dq/ab/2(thetam), thetam/1
  Adding current system noise1/1(idq_physical) -> idq_meas/1, dq/ab/1(dq)

== system EKF_SPM_Slx2019/SUBMOTOR 2/dq//ab1 ==
  dq : Inport
  thetam : Inport  Port=2
  Demux : Demux  Outputs=2
  Gain : Gain  Gain=-1
  Mux : Mux  Inputs=2
  Product{,1..3} (4 alike) : Product  RndMeth=Zero
  Sum : Sum  SaturateOnIntegerOverflow=on  InputSameDT=on  OutDataTypeStr=Inherit: Same as first input
  Sum1 : Sum  Inputs=-+  SaturateOnIntegerOverflow=on  InputSameDT=on  OutDataTypeStr=Inherit: Same as first input
  Trigonometric Function : Trigonometry  Operator=cos
  Trigonometric Function1 : Trigonometry
  ab : Outport
  wires:
  Product3/1 -> Sum1/2
  Product2/1 -> Sum1/1
  Product1/1 -> Sum/2
  Trigonometric Function1/1 -> Product2/2, Product1/2
  Demux/2 -> Product3/1, Product1/1
  Product/1 -> Sum/1
  Trigonometric Function/1 -> Product3/2, Product/2
  Demux/1 -> Product/1, Product2/1
  Sum1/1 -> Mux/2
  Sum/1 -> Mux/1
  Gain/1 -> Trigonometric Function1/1, Trigonometric Function/1
  thetam/1 -> Gain/1
  dq/1 -> Demux/1
  Mux/1 -> ab/1

== system EKF_SPM_Slx2019/Subsystem/ADC-RDC Resolver Continuos TF ==
  note: This zero older hold is kept sampling at the simulation step rate...so it goes with the simulation Runge Kutta
  InputAngle : Inport
  Compensator : TransferFcn  Numerator=[t*(1+a) 2*(1-a)]  Denominator=[t*(1+b) 2*(1-b)]
  Cont Integrator : TransferFcn  Numerator=[c*t 2*c]  Denominator=[2*t 0]
  Cont Integrator1 : TransferFcn  Numerator=[c*t 2*c]  Denominator=[2*t 0]
  Discrete Derivative : simulink/Discrete/Discrete Derivative  gainval=1.0  ICPrevScaledInput=0.0  OutMin=[]  OutMax=[]  OutDataType=fixdt(1, 16)  OutScaling=2^-10  DoSatur=off
  Gain6 : Gain  Gain=k1*k2
  Scope : Scope
  Sum2 : Sum  Inputs=|+-
  Zero-Order Hold : ZeroOrderHold  SampleTime=2.5e-6
  Out Meas Feedback Angle : Outport
  Out Meas Feedback Speed : Outport  Port=2
  wires:
  Cont Integrator/1 -> Compensator/1
  Sum2/1 -> Gain6/1
  Compensator/1 -> Cont Integrator1/1
  InputAngle/1 -> Sum2/1
  Gain6/1 -> Cont Integrator/1
  Discrete Derivative/1 -> Out Meas Feedback Speed/1
  Cont Integrator1/1 -> Scope/1, Zero-Order Hold/1, Out Meas Feedback Angle/1, Sum2/2
  Zero-Order Hold/1 -> Discrete Derivative/1

== system EKF_SPM_Slx2019/Subsystem/NOISE-ADDITION ==
  clean angle : Inport
  clean speed : Inport  Port=2
  Additional Noise generator : Subsystem
  Scope : Scope  NumInputPorts=2
  Sum1 : Sum  Inputs=|++
  Sum3 : Sum  Inputs=++|
  noisy_angle : Outport
  noisy_speed : Outport  Port=2
  wires:
  Additional Noise generator/1(angle_noise) -> Sum3/2
  Sum3/1 -> noisy_angle/1
  Additional Noise generator/2(speed_noise) -> Sum1/1
  clean speed/1 -> Scope/2, Sum1/2
  Sum1/1 -> Scope/1, noisy_speed/1
  clean angle/1 -> Sum3/1

== system EKF_SPM_Slx2019/SUBMOTOR 2/Current Feedback - Second Motor/CURRENT - NOISE ==
  Process Noise : simulink/Sources/Band-Limited White Noise  Cov=ivar*Ts  Ts=Ts  seed=[23341]
  Process Noise1 : simulink/Sources/Band-Limited White Noise  Cov=ivar*Ts  Ts=Ts  seed=[23345]
  Process Noise2 : simulink/Sources/Band-Limited White Noise  Cov=ivar*Ts  Ts=Ts  seed=[23340]
  To Workspace : ToWorkspace  VariableName=Anoise_Motor2  SaveFormat=Timeseries  SampleTime=-1
  To Workspace1 : ToWorkspace  VariableName=Bnoise_Motor2  SaveFormat=Timeseries  SampleTime=-1
  noise_IA : Outport
  noise_IB : Outport  Port=2
  noise_IC : Outport  Port=3
  wires:
  Process Noise/1 -> To Workspace/1, noise_IA/1
  Process Noise2/1 -> noise_IC/1
  Process Noise1/1 -> To Workspace1/1, noise_IB/1

== system EKF_SPM_Slx2019/SUBMOTOR 2/Current Feedback - Second Motor/Clarke3 ==
  ia : Inport
  ib : Inport  Port=2
  ic : Inport  Port=3
  " " : Gain  Gain=2/3  SaturateOnIntegerOverflow=on  OutDataTypeStr=Inherit: Same as input  ParamDataTypeStr=Inherit: Same as input
  "   " : Gain  Gain=1/3  SaturateOnIntegerOverflow=on  OutDataTypeStr=Inherit: Same as input  ParamDataTypeStr=Inherit: Same as input
  "    " : Gain  Gain=1/3  SaturateOnIntegerOverflow=on  OutDataTypeStr=Inherit: Same as input  ParamDataTypeStr=Inherit: Same as input
  " 1/root3" : Gain  Gain=0.57735026918962576450914878050196  SaturateOnIntegerOverflow=on  OutDataTypeStr=Inherit: Same as input  ParamDataTypeStr=Inherit: Same as input
  Sum1 : Sum  Inputs=+-  SaturateOnIntegerOverflow=on  InputSameDT=on  OutDataTypeStr=Inherit: Same as first input
  Sum4 : Sum  Inputs=+--  SaturateOnIntegerOverflow=on  InputSameDT=on  OutDataTypeStr=Inherit: Same as first input
  ialpha : Outport
  ibeta : Outport  Port=2
  wires:
  Sum4/1 -> ialpha/1
  " "/1 -> Sum4/1
  ia/1 -> " "/1
  "    "/1 -> Sum4/2
  "   "/1 -> Sum4/3
  ib/1 -> "    "/1, Sum1/1
  ic/1 -> "   "/1, Sum1/2
  Sum1/1 -> " 1/root3"/1
  " 1/root3"/1 -> ibeta/1

== system EKF_SPM_Slx2019/SUBMOTOR 2/Current Feedback - Second Motor/Zero noise ==
  Constant : Constant  Value=0
  Constant4 : Constant  Value=0
  Constant5 : Constant  Value=0
  Out1 : Outport
  Out2 : Outport  Port=2
  Out3 : Outport  Port=3
  wires:
  Constant/1 -> Out2/1
  Constant4/1 -> Out3/1
  Constant5/1 -> Out1/1

== system EKF_SPM_Slx2019/SUBMOTOR 2/Current_Controller/Emulate Measurement noise on dq axis ==
  Constant : Constant  Value=seed_5
  Constant1 : Constant  Value=0
  Constant2 : Constant  Value=sqrt(R_cov(1,1))
  Constant3 : Constant  Value=seed_4
  Constant4 : Constant  Value=sqrt(R_cov(2,2))
  MATLAB Function : MATLAB Function  TreatAsAtomicUnit=on
  MATLAB Function1 : MATLAB Function  TreatAsAtomicUnit=on
  Zero-Order Hold : ZeroOrderHold  SampleTime=Ts
  Zero-Order Hold1 : ZeroOrderHold  SampleTime=Ts
  Out1 : Outport
  Out2 : Outport  Port=2
  wires:
  Constant1/1 -> MATLAB Function1/1(mean), MATLAB Function/1(mean)
  Constant3/1 -> MATLAB Function/3(s1)
  Constant/1 -> MATLAB Function1/3(s1)
  Zero-Order Hold/1 -> Out1/1
  Constant4/1 -> MATLAB Function1/2(stdDev)
  MATLAB Function/1(y) -> Zero-Order Hold/1
  Zero-Order Hold1/1 -> Out2/1
  MATLAB Function1/1(y) -> Zero-Order Hold1/1
  Constant2/1 -> MATLAB Function/2(stdDev)

== system EKF_SPM_Slx2019/SUBMOTOR 2/HealthySUbmotor - PI//1/Adding angle system noise ==
  theta_ideal : Inport
  Constant : Constant  Value=0
  Manual Switch : ManualSwitch  CurrentSetting=0
  Sum1 : Sum
  sys_noise : simulink/Sources/Band-Limited White Noise  Cov=[Q(1,1)*Ts]  Ts=Ts  seed=[seed_6]
  tehta_physical : Outport
  wires:
  Constant/1 -> Manual Switch/2
  Manual Switch/1 -> Sum1/2
  Sum1/1 -> tehta_physical/1
  sys_noise/1 -> Manual Switch/1
  theta_ideal/1 -> Sum1/1

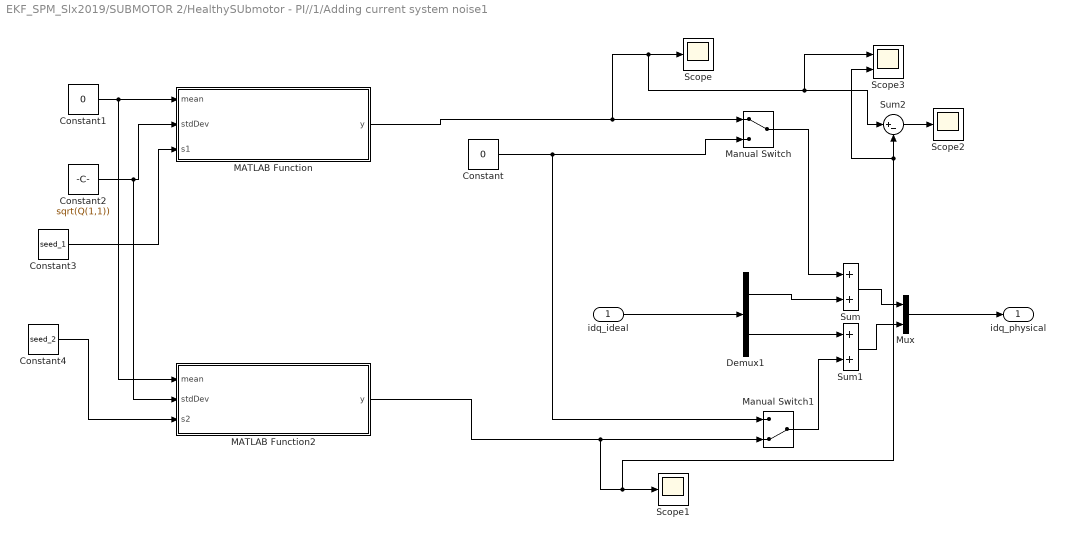
== system EKF_SPM_Slx2019/SUBMOTOR 2/HealthySUbmotor - PI//1/Adding current system noise1 ==
  idq_ideal : Inport
  Constant : Constant  Value=0
  Constant1 : Constant  Value=0
  Constant2 : Constant  Value=sqrt(Q(1,1))
  Constant3 : Constant  Value=seed_1
  Constant4 : Constant  Value=seed_2
  Demux1 : Demux  Outputs=2
  MATLAB Function : MATLAB Function  TreatAsAtomicUnit=on
  MATLAB Function2 : MATLAB Function  TreatAsAtomicUnit=on
  Manual Switch : ManualSwitch
  Manual Switch1 : ManualSwitch  CurrentSetting=0
  Mux : Mux  Inputs=2
  Scope : Scope
  Scope1 : Scope
  Scope2 : Scope
  Scope3 : Scope  NumInputPorts=2
  Sum : Sum
  Sum1 : Sum
  Sum2 : Sum  Inputs=|+-
  idq_physical : Outport
  wires:
  Demux1/2 -> Sum1/1
  idq_ideal/1 -> Demux1/1
  Sum1/1 -> Mux/2
  Demux1/1 -> Sum/2
  Sum/1 -> Mux/1
  Mux/1 -> idq_physical/1
  MATLAB Function/1(y) -> Scope3/1, Sum2/1, Scope/1, Manual Switch/1
  Constant/1 -> Manual Switch1/1, Manual Switch/2
  Manual Switch1/1 -> Sum1/2
  Manual Switch/1 -> Sum/1
  Constant1/1 -> MATLAB Function2/1(mean), MATLAB Function/1(mean)
  Constant2/1 -> MATLAB Function2/2(stdDev), MATLAB Function/2(stdDev)
  MATLAB Function2/1(y) -> Scope3/2, Sum2/2, Scope1/1, Manual Switch1/2
  Constant3/1 -> MATLAB Function/3(s1)
  Constant4/1 -> MATLAB Function2/3(s2)
  Sum2/1 -> Scope2/1

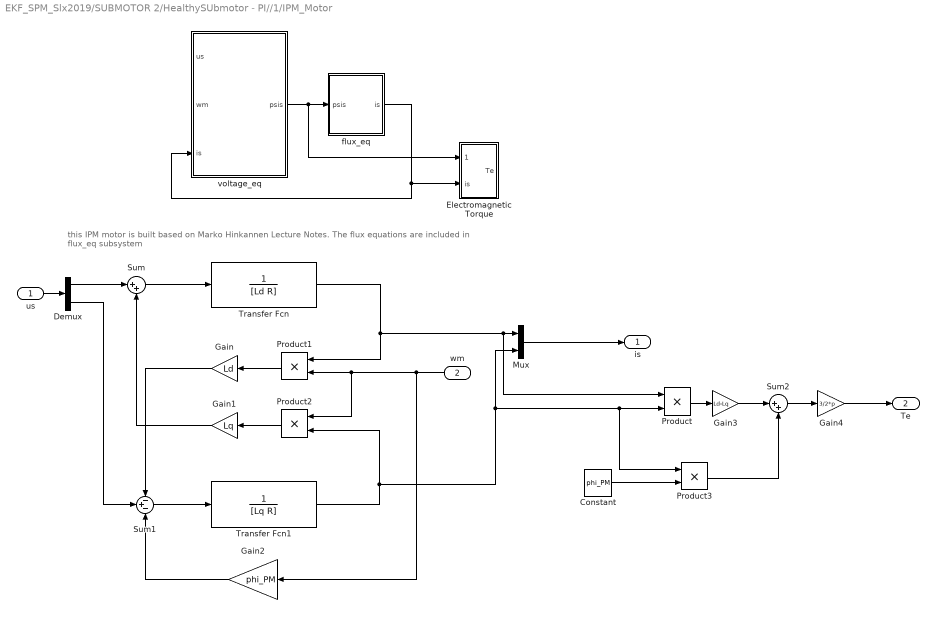
== system EKF_SPM_Slx2019/SUBMOTOR 2/HealthySUbmotor - PI//1/IPM_Motor ==
  note: this IPM motor is built based on Marko Hinkannen Lecture Notes. The flux equations are included in flux_eq subsystem
  us : Inport
  wm : Inport  Port=2
  Constant : Constant  Value=phi_PM
  Demux : Demux  Outputs=2
  Electromagnetic Torque : Subsystem
  Gain : Gain  Gain=Ld
  Gain1 : Gain  Gain=Lq
  Gain2 : Gain  Gain=phi_PM
  Gain3 : Gain  Gain=Ld-Lq
  Gain4 : Gain  Gain=3/2*p
  Mux : Mux  Inputs=2
  Product{,1..3} (4 alike) : Product
  Sum : Sum  Inputs=|++
  Sum1 : Sum  Inputs=-+-
  Sum2 : Sum  Inputs=|++
  Transfer Fcn : TransferFcn  Denominator=[Ld R]
  Transfer Fcn1 : TransferFcn  Denominator=[Lq R]
  flux_eq : Subsystem
  voltage_eq : Subsystem
  is : Outport
  Te : Outport  Port=2
  wires:
  flux_eq/1(is) -> Electromagnetic Torque/2(is), voltage_eq/3(is)
  voltage_eq/1(psis) -> Electromagnetic Torque/1(psis), flux_eq/1(psis)
  us/1 -> Demux/1
  Demux/1 -> Sum/1
  Sum/1 -> Transfer Fcn/1
  Transfer Fcn/1 -> Product/1, Mux/1, Product1/1
  wm/1 -> Gain2/1, Product2/1, Product1/2
  Product1/1 -> Gain/1
  Product2/1 -> Gain1/1
  Gain1/1 -> Sum/2
  Gain/1 -> Sum1/1
  Sum1/1 -> Transfer Fcn1/1
  Demux/2 -> Sum1/2
  Transfer Fcn1/1 -> Product2/2, Product3/1, Product/2, Mux/2
  Gain2/1 -> Sum1/3
  Mux/1 -> is/1
  Product/1 -> Gain3/1
  Gain3/1 -> Sum2/1
  Sum2/1 -> Gain4/1
  Product3/1 -> Sum2/2
  Gain4/1 -> Te/1
  Constant/1 -> Product3/2

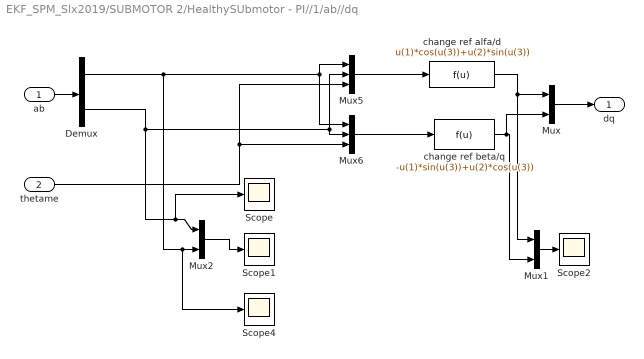
== system EKF_SPM_Slx2019/SUBMOTOR 2/HealthySUbmotor - PI//1/ab//dq ==
  ab : Inport
  thetame : Inport  Port=2
  Demux : Demux  Outputs=2
  Mux : Mux  Inputs=2
  Mux1 : Mux  Inputs=2
  Mux2 : Mux  Inputs=2
  Mux5 : Mux  Inputs=3
  Mux6 : Mux  Inputs=3
  Scope{,1..2,4} (4 alike) : Scope
  change ref alfa/d : Fcn  Expr=u(1)*cos(u(3))+u(2)*sin(u(3))
  change ref beta/q : Fcn  Expr=-u(1)*sin(u(3))+u(2)*cos(u(3))
  dq : Outport
  wires:
  Demux/1 -> Scope4/1, Mux2/2, Mux5/1, Mux6/1
  Demux/2 -> Scope/1, Mux2/1, Mux6/2, Mux5/2
  thetame/1 -> Mux6/3, Mux5/3
  change ref alfa/d/1 -> Mux/1, Mux1/1
  change ref beta/q/1 -> Mux/2, Mux1/2
  Mux2/1 -> Scope1/1
  Mux1/1 -> Scope2/1
  ab/1 -> Demux/1
  Mux/1 -> dq/1
  Mux5/1 -> change ref alfa/d/1
  Mux6/1 -> change ref beta/q/1

== system EKF_SPM_Slx2019/SUBMOTOR 2/HealthySUbmotor - PI//1/dq//ab ==
  dq : Inport
  thetam : Inport  Port=2
  Demux : Demux  Outputs=2
  Gain : Gain  Gain=-1
  Mux : Mux  Inputs=2
  Product{,1..3} (4 alike) : Product  RndMeth=Zero
  Sum : Sum  SaturateOnIntegerOverflow=on  InputSameDT=on  OutDataTypeStr=Inherit: Same as first input
  Sum1 : Sum  Inputs=-+  SaturateOnIntegerOverflow=on  InputSameDT=on  OutDataTypeStr=Inherit: Same as first input
  Trigonometric Function : Trigonometry  Operator=cos
  Trigonometric Function1 : Trigonometry
  ab : Outport
  wires:
  Product3/1 -> Sum1/2
  Product2/1 -> Sum1/1
  Product1/1 -> Sum/2
  Trigonometric Function1/1 -> Product2/2, Product1/2
  Demux/2 -> Product3/1, Product1/1
  Product/1 -> Sum/1
  Trigonometric Function/1 -> Product3/2, Product/2
  Demux/1 -> Product/1, Product2/1
  Sum1/1 -> Mux/2
  Sum/1 -> Mux/1
  Gain/1 -> Trigonometric Function1/1, Trigonometric Function/1
  thetam/1 -> Gain/1
  dq/1 -> Demux/1
  Mux/1 -> ab/1

== system EKF_SPM_Slx2019/Subsystem/NOISE-ADDITION/Additional Noise generator ==
  Constant4 : Constant  Value=snoise_mean
  Constant5 : Constant  Value=snoise_std
  LSB angle : Gain  Gain=gainAngle_noise
  LSB speed : Gain  Gain=gainSpeed_noise
  Scope2 : Scope
  ZOH speed - Speed Loop1 : ZeroOrderHold  SampleTime=Tspeed
  ZOH speed - Speed Loop2 : ZeroOrderHold  SampleTime=Tspeed
  generation of discrete values for gauss noise : MATLAB Function  TreatAsAtomicUnit=on
  angle_noise : Outport
  speed_noise : Outport  Port=2
  wires:
  Constant5/1 -> ZOH speed - Speed Loop2/1
  Constant4/1 -> ZOH speed - Speed Loop1/1
  ZOH speed - Speed Loop1/1 -> generation of discrete values for gauss noise/1(mean)
  generation of discrete values for gauss noise/1(y) -> LSB angle/1, Scope2/1, LSB speed/1
  ZOH speed - Speed Loop2/1 -> generation of discrete values for gauss noise/2(stdDev)
  LSB speed/1 -> speed_noise/1
  LSB angle/1 -> angle_noise/1

== system EKF_SPM_Slx2019/SUBMOTOR 2/HealthySUbmotor - PI//1/IPM_Motor/Electromagnetic Torque ==
  psis : Inport
  is : Inport  Port=2
  Fcn : Fcn  Expr=u(1)*u(4) - u(2)*u(3)
  Gain : Gain  Gain=3/2*p
  Mux : Mux  Inputs=2
  Te : Outport
  wires:
  Gain/1 -> Te/1
  is/1 -> Mux/2
  psis/1 -> Mux/1
  Mux/1 -> Fcn/1
  Fcn/1 -> Gain/1

== system EKF_SPM_Slx2019/SUBMOTOR 2/HealthySUbmotor - PI//1/IPM_Motor/flux_eq ==
  psis : Inport
  Gain : Gain  Gain=Linv  Multiplication=Matrix(K*u) (u vector)
  Gain1 : Gain  Gain=d
  Sum : Sum  Inputs=|++
  phi_PM : Constant  Value=phi_PM
  is : Outport
  wires:
  psis/1 -> Gain/1
  phi_PM/1 -> Gain1/1
  Gain/1 -> Sum/1
  Gain1/1 -> Sum/2
  Sum/1 -> is/1

== system EKF_SPM_Slx2019/SUBMOTOR 2/HealthySUbmotor - PI//1/IPM_Motor/voltage_eq ==
  us : Inport
  wm : Inport  Port=2
  is : Inport  Port=3
  Gain : Gain  Gain=Rs
  Gain1 : Gain  Gain=J  Multiplication=Matrix(K*u) (u vector)
  Integrator : Integrator
  Product : Product
  Sum : Sum  Inputs=|+-
  Sum1 : Sum  Inputs=|+-
  psis : Outport
  wires:
  Integrator/1 -> Gain1/1, psis/1
  Gain/1 -> Sum/2
  Sum1/1 -> Integrator/1
  us/1 -> Sum/1
  wm/1 -> Product/2
  Product/1 -> Sum1/2
  is/1 -> Gain/1
  Sum/1 -> Sum1/1
  Gain1/1 -> Product/1

== matlab function EKF_SPM_Slx2019/Adaptive Extended Kalman Filter ==
  data: xe input size=[4,1]; u input size=[2,1]; y input size=[2,1]; xe output; Ld parameter; Lq parameter; R parameter; R_cov parameter; Ts parameter; phi_PM parameter; P input size=[4,4]; Pout output size=[4,4]; Qd parameter; vout output; Cout output; yout output; Kout output
function [xe, Pout, vout,Cout,yout,Kout] = AEFK(xe, u,y, Ld, Lq, R, R_cov, Ts, phi_PM, P, Qd)
% [xe, Pout, Qout] = AEFK(xe, u,y, Ld, Lq, R, R_cov, Ts, phi_PM, P, Qd)
% NC extended kalman filter function

% adaptive extended kalman filter version (assuming R constant and only Q not known)

% adaptive parameters --------------
N = 10; % window length

persistent v;
if isempty(v)
    v = zeros(2,N);
end

persistent C;
if isempty(C)
    C = zeros(2,2);
end

% NC extended kalman filter function for SPM

R_cov = R;
%Qd = Qd*100;

L = Ld;

% input -------------------------------------------------------------------
% getting the estimate
ia = xe(1);
ib = xe(2);
we = xe(3);
theta = xe(4);

G = [1/L 0 0 0; ...
    0 1/L 0 0 ]';

H = [1 0 0 0; ...
    0 1 0 0];

f = [-R/L*ia + we*phi_PM/L*sin(theta) ; ...
    -R/L*ib - we*phi_PM/L*cos(theta) ; ...
    0 ; ...
    we];

% Jacobian matrix
F11 = -R/Ld;
F13 = phi_PM/L*sin(theta);
F14 = phi_PM*we/L*cos(theta);
F22 = -R/L;
F23 = -phi_PM/L*cos(theta);
F24 = phi_PM*we/L*sin(theta);
F43 = 1;

F = [F11 0 F13 F14; ...
    0 F22 F23 F24 ; ...
    0 0 0 0 ; ...
    0 0 F43 0];

phid = eye(4) + Ts*F; % state matrix

% Prediction
xe = xe + (f + G*u)*Ts;
%xe = phid*xe + G*u*Ts;

% xe(1) = (1-R/L*Ts)*xe(1) + xe(3)*phi_PM*sin(xe(4))/L + Ts/L*u(1);
% xe(2) = (1-R/L*Ts)*xe(2) - xe(3)*phi_PM*cos(xe(4))/L + Ts/L*u(2);
% xe(3) = xe(3);
% xe(4) = xe(4) + xe(3)*Ts;

P = phid*P*phid' + Qd;
%P = P + (F*P + P*F')*Ts + Qd;
%xe(4) = bound_angle(xe(4)); % bound angle

% Kalman gain 
Cc = P*H';
K = Cc*(H*Cc+R_cov)^(-1);
Kout = K;

% observation
v(:,1) = y-H*xe; % innovation residual with respect to measurement
xe = xe + K*v(:,1);
%Pout = (eye(4)-K*H)*P;
Pout = (eye(4)-K*H)*P*(eye(4)-K*H)' + K*R_cov*K'; % covariance correction Joseph' equation

xe(4) = bound_angle(xe(4)); % bound angle

%% Covariance matrix update (adaptation step) 

yout = y;
% residual matrix sum (to be vectorized)
for j = 1:N
    C = C + v(:,j)*v(:,j)';
end
C = C/N;

% output stuff
Cout = C;
vout = v;

% update history
for j = N:-1:2
    v(:,j) = v(:,j-1);
end

% update covariance matrix
%Qout = K*C*K'; %Q

% TO DO: we need to go into an SVD situation for getting the nearest
% positive definite equation
% =========================================================================


%% computation with method given in Improving Adaptive Kalman Estimation in GPS/INS integration
% alpha = trace(H*(phid*P*phid' + Qd)*H')/...
%     trace();

Qout = Qd;

end

% extra functions

function angle = bound_angle(angle)
% keep it bounded in its true range

if (angle<0)
    angle = -angle;
end

while (angle >= 2*pi)
    angle = angle - 2*pi;
end

end

== matlab function EKF_SPM_Slx2019/SUBMOTOR 2/MATLAB Function ==
  data: mi output; u input; y output; Vdc input; a output
function [mi,y,a] = limiter(u,Vdc)

valpha = u(1);
vbeta = u(2);


m = hypot(valpha,vbeta);

mi = m/(2/pi*Vdc);

a = atan2(vbeta,valpha);

y = u;

== matlab function EKF_SPM_Slx2019/SUBMOTOR 2/Basic digital controller and AntiWindup ==
  data: id_ref input; iq_ref input; is input; yd output; yq output; Ts parameter; Id_new output; kp parameter; ki parameter; Id input; Iq input; Lq parameter; Ld parameter; Iq_new output; Vdc parameter; wm input; thetas input; id output; iq output; measNoise_d input; measNoise_q input; mi output
function [yd,yq,Id_new, Iq_new,id,iq,mi] = Controller_implementation(id_ref,iq_ref,is,Ts,kp, ...
                                            ki,Id,Iq, Lq,Ld,Vdc, wm,thetas,measNoise_d,measNoise_q)

persistent awd
if isempty(awd)
    awd = 0;
end
persistent awq
if isempty(awq)
    awq = 0;
end

if ~iscolumn(is)
    is = is';
end

%% Current controller 

% current split
ialpha = is(1);
ibeta = is(2);

%% angle adjustment for the second motor
% (for the second sub-motor we need to make a shift of pi/6)
% park transform of the feedback
co = cos(thetas);
si = sin(thetas);
id = co*ialpha + si*ibeta;
iq = -si*ialpha + co*ibeta;

% adding noise
id = id + measNoise_d;
iq = iq + measNoise_q;

%% errors
ed = id_ref - id;
eq = iq_ref - iq;

%% PI controller
ud = kp*ed + ki*Ts*Id;    % prop
uq = kp*eq + ki*Ts*Iq;    % prop

% compensation
ud_comp = ud -Lq*wm*iq;
uq_comp = uq +Ld*wm*id;

% Delay compensation
thetasc = thetas + 1*Ts*wm;   % discrete-time delays
uss_ref = (ud_comp + 1i*uq_comp) * exp(1j*thetasc); % compensation

%% Preparing valpha - vbeta for SVM - with saturation 
% Components of the voltage space vector
ualpha_ref = real(uss_ref);
ubeta_ref  = imag(uss_ref);

% maximum modulation index for the power converter (SVM implementation 
% according to Lee: A novel overmodulation technique for spece vector PWM Inverters)
uss_abs = hypot(ubeta_ref,ualpha_ref);
mi = uss_abs/(2/pi*Vdc);

% clamping and building reference in alpha-beta frame
if mi >= 1 
    uss_abs = 2/pi*Vdc;
    phase_ref = atan2(ualpha_ref,ubeta_ref);
    uss_ref_lim = uss_abs*(cos(phase_ref) + 1j*sin(phase_ref))*0.995; % extra safety
else
    uss_ref_lim = uss_ref;
end

% In estimated rotor flux coordinates
us_ref_lim = exp(-1j*thetasc)*uss_ref_lim; 

% back to real dq
yd = real(us_ref_lim);
yq = imag(us_ref_lim);


%% ANTI WINDUP SATURATION

% % limit
% limit = 2/pi*Vdc*0.98;
% 
% % magnitude of the reference vector
% u_ref = sqrt(ud_comp^2+uq_comp^2);
% 
% % clamping with reference to the modulation index (same as the space vector modulation)
% if ( u_ref >=  limit)
%     ratio = limit/u_ref;
%     yd = ud_comp*ratio;
%     yq = uq_comp*ratio;
% else
%     yd = ud_comp;
%     yq = uq_comp;
% end
% 
% %y_mag = sqrt(yd^2+yq^2); % this is just for checking
% 
% back calc done here:
awd = 1/kp*(yd - ud_comp);
awq = 1/kp*(yq - uq_comp);

Id_new = Id + (ed+awd);        % integral
Iq_new = Iq + (eq+awq);        % integral



end

== matlab function EKF_SPM_Slx2019/Subsystem/limit 0 - 360 ==
  data: u input; y output
function y = adjust_angle(u)

% keep it bounded in its true range
while (u >= 2*pi)
    u = u - 2*pi;
end

y = u;

== matlab function EKF_SPM_Slx2019/SUBMOTOR 2/Current_Controller/Emulate Measurement noise on dq axis/MATLAB Function ==
  data: mean input; y output; stdDev input; s1 input
function y  = white_gauss_noise(mean,stdDev,s1)

% NC generation of gauss white noise with the simulation period (not sampling period)

% defining the seed of interest for this simulation
persistent first_fcn_call
if isempty(first_fcn_call)
    rand('seed',s1);
    first_fcn_call = 0;
end

spare = 0;
hasSpare = 0;

if(hasSpare)
    hasSpare = 0;
    y = spare*stdDev + mean;
else
    % init var for loops
    s = 0; u = 0; v = 0;
    while(s >= 1.0 || s == 0)
        u = rand * 2.0 - 1.0;
        v = rand * 2.0 - 1.0;        
        s = u^2+v^2;
    end
    s = sqrt(-2.0*log(s)/s);
    spare = v*s;
    hasSpare = 1;
    y = mean + stdDev*u*s;
end

== matlab function EKF_SPM_Slx2019/Subsystem/NOISE-ADDITION/Additional Noise generator/generation of discrete values for gauss noise ==
  data: mean input; y output; stdDev input
function y = white_gauss_noise(mean,stdDev)

% white_gauss_noise - function can store the simulation

spare = 0;
hasSpare = 0;

if (hasSpare) 
    
    hasSpare = 0;
    y = spare * stdDev + mean; 

else
    % init vars for loop
    s = 0; u = 0; v = 0;
    while (s >= 1.0 || s == 0.0)
%             u = (rand() / ((double)RAND_MAX)) * 2.0 - 1.0;
%             v = (rand() / ((double)RAND_MAX)) * 2.0 - 1.0;

        u = rand * 2.0 - 1.0;
        v = rand * 2.0 - 1.0;

        s = u^2 + v^2;
        
    end
    s = sqrt(-2.0 * log(s) / s);
    spare = v * s;
    hasSpare = 1;
    y = mean + stdDev * u * s;

end

% Discrete rounding
y = round(y);
